simulink model "Lab6_PartA"  (R2025b)
settings: Solver=VariableStepAuto  StartTime=0.0  StopTime=20  RelTol=1e-12
settings Model: Creator=Murl0  LastModifiedBy=Murl0

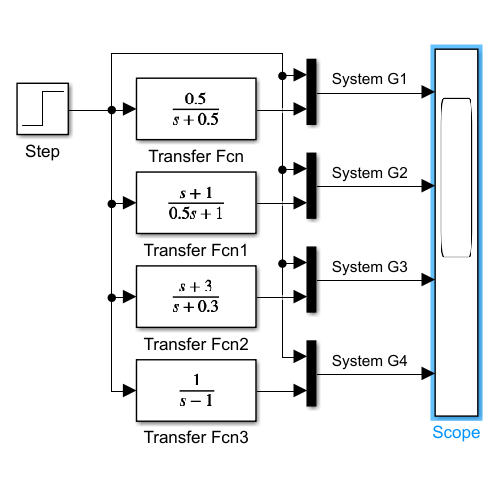
[thumbnail: Simulink's stored preview of the top-level diagram]
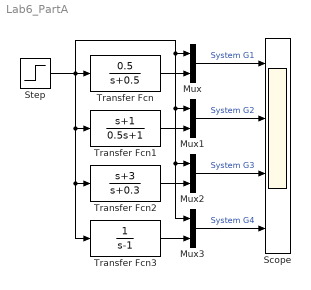
== system Lab6_PartA ==
  Mux{,1..3} (4 alike) : Mux  Inputs=2
  Scope : Scope  NumInputPorts=4
      settings: ActiveDisplayYMinimum=-0.12499999999999997  ActiveDisplayYMaximum=1.125
  Step : Step  SampleTime=0
  Transfer Fcn : TransferFcn  Numerator=[0.5]  Denominator=[1 0.5]
  Transfer Fcn1 : TransferFcn  Numerator=[1 1]  Denominator=[0.5 1]
  Transfer Fcn2 : TransferFcn  Numerator=[1 3]  Denominator=[1 0.3]
  Transfer Fcn3 : TransferFcn  Denominator=[1 -1]
  wires:
  Transfer Fcn/1 -> Mux/2
  Step/1 -> Transfer Fcn3/1, Transfer Fcn2/1, Transfer Fcn1/1, Transfer Fcn/1, Mux3/1, Mux2/1, Mux1/1, Mux/1
  Transfer Fcn1/1 -> Mux1/2
  Transfer Fcn2/1 -> Mux2/2
  Transfer Fcn3/1 -> Mux3/2
  Mux/1 -> Scope/1  "System G1"
  Mux1/1 -> Scope/2  "System G2"
  Mux2/1 -> Scope/3  "System G3"
  Mux3/1 -> Scope/4  "System G4"
